simulink model "nimp"  (R2016a)
settings: Solver=VariableStepAuto  StartTime=0.0  StopTime=1e5  RelTol=1e-3
libraries: simCryogenics_lib x10, nesl_utility x5
settings Model: Creator=FB229602  LastModifiedBy=FB229602
settings SimscapeCC: SimscapeLogType=all

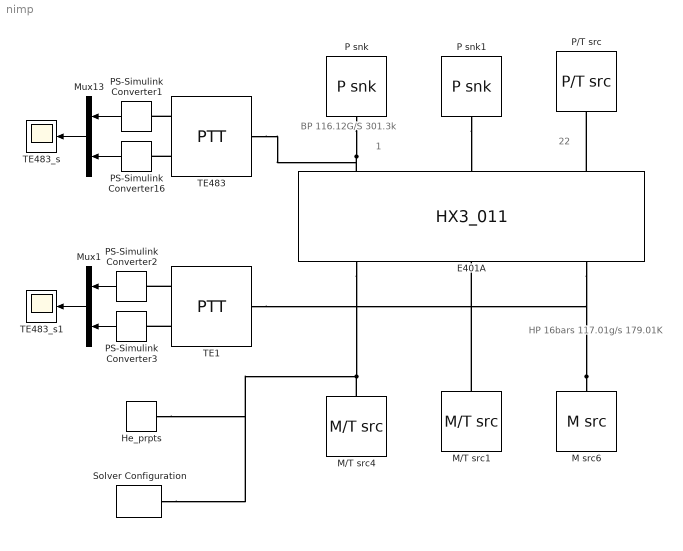
== system nimp ==
  note: 22
  note: 1
  note: BP
      | 116.12G/S
      | 301.3k
  note: HP
      | 16bars
      | 117.01g/s
      | 179.01K
  E401A : simCryogenics_lib/Elements/HX3_011  N=9  Vh=0.118 m^3  Vm=0.055 m^3  Vc=0.008 km^3  M=281 kg  Kh=0.062/0.11612 s*bar/kg  Km=0.033/0.11701 s*bar/kg  Kc=0.021/.0026 s*bar/kg  hh_m=1 J/s/K  hh_c=6e4 J/s/K  hm_c=500 J/s/K  Th0=300 K  Ph0=16 bar  Mh0=0.11612 kg/s  Tm0=179 K  Pm0=1 bar  Mm0=0.002 kg/s  Tc0=179 K  Pc0=1.05 bar  Mc0=0.116 kg/s  sensh=0  sensm=1  sensc=1
  He_prpts : simCryogenics_lib/Utilities/He_prpts  P_min=0.1 bar  P_max=30 bar  T_min=3 K  T_max=320 K  N=100  Mol=4.0026 * 10 ^ (- 3) kg/mol
  M src6 : simCryogenics_lib/Sources_Sinks/M src  M=0.116 kg/s
  M/T src1 : simCryogenics_lib/Sources_Sinks/M//T src  M=0.00000026 kg/s  T=179 K
  M/T src4 : simCryogenics_lib/Sources_Sinks/M//T src  M=0.116 kg/s  T=179 K
  Mux1 : Mux  Inputs=2
  Mux13 : Mux  Inputs=2
  P snk : simCryogenics_lib/Sources_Sinks/P snk  P=1.05 bar
  P snk1 : simCryogenics_lib/Sources_Sinks/P snk  P=1.05 bar
  P/T src : simCryogenics_lib/Sources_Sinks/P//T src  P=14.73 bar  T=305 K
  PS-Simulink Converter{1..3,16} (4 alike) : nesl_utility/PS-Simulink Converter  PhysicalDomain=network_engine_domain  SubClassName=ps_output  LeftPortType=input  RightPortType=output  PseudoPeriodic=off  Frequencies=[]  Unit=1  AffineConversion=off
  Solver Configuration : nesl_utility/Solver Configuration  PhysicalDomain=network_engine_domain  SubClassName=solver  LeftPortType=input  RightPortType=generic  Accelerate=off  Tones=[]  Harmonics=[]  SimulateNoise=off  Profile=off  UseLocalSampling=off  EnableSwitchedLinearOptims=on  FrequencyDomain=off  UseCCode=off  RelTol=0.001  AbsTol=1e-06  MinStep=1e-09  ToWorkspace=off  RevertToSquareIcSolve=off  NumHomotopyIterations=100  PhasorMode=off  PhasorModeNumHarmonics=1  OverrideAbsTol=off  DoDC=off  ResidualTolerance=1e-09  UseLocalSolver=off  LocalSolverChoice=NE_BACKWARD_EULER_ADVANCER  LocalSolverSampleTime=0.001  DoFixedCost=off  MaxNonlinIter=3  MaxModeIter=2  LinearAlgebra=Sparse  DelaysMemoryBudget=1024  AutomaticFiltering=on  FilteringTimeConstant=0.001
  TE1 : simCryogenics_lib/Sensors/PTT
  TE483 : simCryogenics_lib/Sensors/PTT
  TE483_s : Scope
  TE483_s1 : Scope
  wires:
  PS-Simulink Converter16/1 -> Mux13/2
  Mux13/1 -> TE483_s/1
  PS-Simulink Converter1/1 -> Mux13/1
  PS-Simulink Converter3/1 -> Mux1/2
  Mux1/1 -> TE483_s1/1
  PS-Simulink Converter2/1 -> Mux1/1
  connections:
  P snk/RConn1 -- E401A/LConn1 -- TE483/LConn1
  M/T src4/RConn1 -- E401A/RConn1 -- He_prpts/RConn1 -- Solver Configuration/RConn1
  E401A/LConn3 -- P/T src/RConn1
  M src6/RConn1 -- E401A/RConn3 -- TE1/LConn1
  TE483/RConn2 -- PS-Simulink Converter16/LConn1
  TE483/RConn1 -- PS-Simulink Converter1/LConn1
  TE1/RConn2 -- PS-Simulink Converter3/LConn1
  TE1/RConn1 -- PS-Simulink Converter2/LConn1
  M/T src1/RConn1 -- E401A/RConn2
  P snk1/RConn1 -- E401A/LConn2
